simulink model "lagrange_int_1"  (Simulink 7.8)
settings: Solver=ode45  StartTime=0.0  StopTime=1  RelTol=1e-3
values from neighbouring files (symbols this model uses):
  b = fir1(nr-1,0.5)    [adapt_filter1.m]    (also in adapt_filter2.m; analog_tp1.m = zeros(5, nord+1); analog_tp2.m = zeros(5, nord+1))
  L = 24    [G722_1.m]    (also in adaptiv_2.m = length(h); adaptiv_3.m = length(h); audio_test1.m = 64; audio_test2.m = 64)
  Ts = 1/fs    (= 6.25e-05)    [G722_1.m]    (also in adaptiv_2.m = 0.001; adaptiv_3.m = 0.001; adaptiv_4.m = 0.001; adaptiv_5.m = 0.001)
undefined symbols (not defined in the file or in its folder): fb
libraries: dsparch4 x1, dspsigops x1
settings Model: Creator=svenhoffmann  LastModifiedBy=josef  ExtModeAutoUpdateStatusClock=off
settings DataIOCC: SignalLoggingName=sigsOut
settings OptimizationCC: InitFltsAndDblsToZero=on
settings DebuggingCC: SaveWithParameterizedLinksMsg=none  SignalResolutionControl=TryResolveAllWithWarning  SolverPrmCheckMsg=none  MultiTaskDSMMsg=warning  MultiTaskCondExecSysMsg=none  FcnCallInpInsideContextMsg=Use local settings  StrictBusMsg=None
settings HardwareCC: TargetUnknown=on
settings RTWCC: IncludeERTFirstTime=on
settings GRTTargetCC: TargetFcnLib=ansi_tfl_tmw.mat

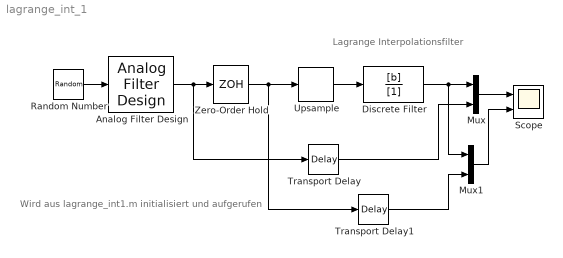
== system lagrange_int_1 ==
  note: Lagrange
      | Interpolationsfilter
  note: Wird aus lagrange_int1.m
      | initialisiert und aufgerufen
  Analog Filter Design : dsparch4/Analog Filter Design  method=Butterworth  filttype=Lowpass  N=8  Wlo=2*pi*fb  Whi=80  Rp=2  Rs=40
  Discrete Filter : DiscreteFilter  Numerator=[b]  Denominator=[1]  SampleTime=Ts/L
  Mux : Mux  Inputs=2
  Mux1 : Mux  Inputs=2
  Random Number : RandomNumber  SampleTime=0
  Scope : Scope  NumInputPorts=2
      settings: YMin=-5~-5  YMax=5~5
  Transport Delay : TransportDelay  DelayTime=0.003
  Transport Delay1 : TransportDelay  DelayTime=0.003
  Upsample : dspsigops/Upsample  N=L  phase=0  InputProcessing=Inherited (this choice will be removed - see release notes)  RateOptions=Allow multirate processing  ic=0  mode=Unused parameter value
  Zero-Order Hold : ZeroOrderHold  SampleTime=Ts
  wires:
  Random Number/1 -> Analog Filter Design/1
  Analog Filter Design/1 -> Zero-Order Hold/1, Transport Delay/1
  Zero-Order Hold/1 -> Upsample/1, Transport Delay1/1
  Upsample/1 -> Discrete Filter/1
  Discrete Filter/1 -> Mux/1, Mux1/1
  Transport Delay/1 -> Mux/2
  Mux/1 -> Scope/1
  Mux1/1 -> Scope/2
  Transport Delay1/1 -> Mux1/2
